simulink model "SimulacionDataReal"  (R2023b)
settings: Solver=ode1be  StartTime=0.0  StopTime=30  FixedStep=0.001  RelTol=1e-3
undefined symbols (not defined in the file): k1, k2, P, W1_0, W2_0
settings Model: Creator=raul  LastModifiedBy=raul
settings OptimizationCC: ReuseModelBlockBuffer=off

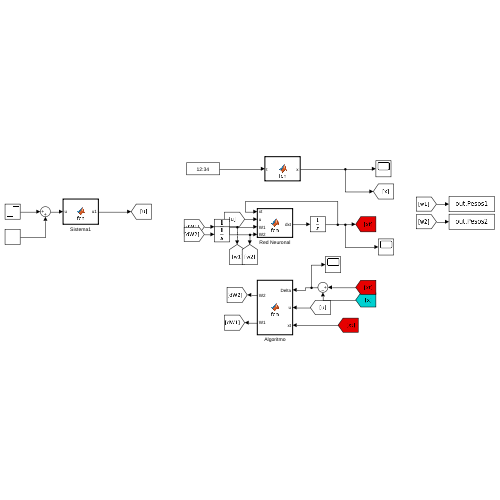
[thumbnail: Simulink's stored preview of the top-level diagram]
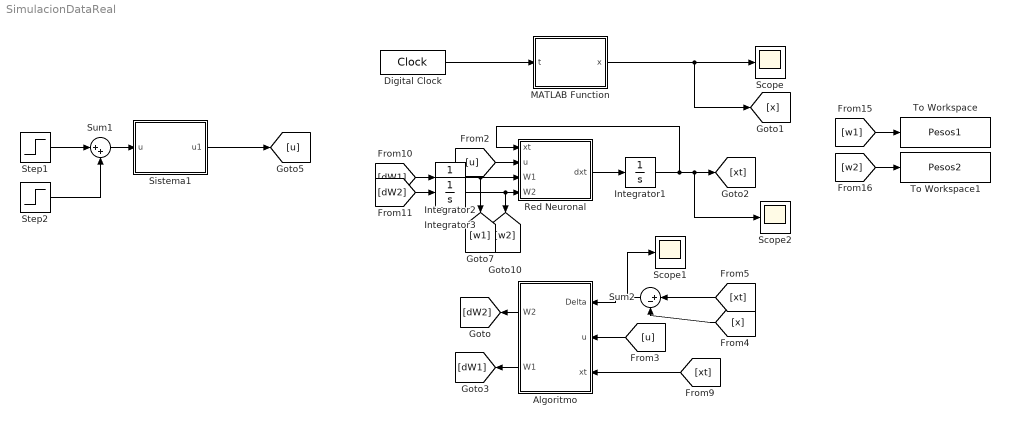
== system SimulacionDataReal ==
  Algoritmo : MATLAB Function  TreatAsAtomicUnit=on
  Digital Clock : DigitalClock  SampleTime=0.01
  Integrator1 : Integrator  InitialCondition=zeros(40,1)
  Integrator2 : Integrator  InitialCondition=W1_0
  Integrator3 : Integrator  InitialCondition=W2_0
  MATLAB Function : MATLAB Function  TreatAsAtomicUnit=on
  Red Neuronal : MATLAB Function  TreatAsAtomicUnit=on
  Scope : Scope
  Scope1 : Scope
  Scope2 : Scope
  Sistema1 : MATLAB Function  TreatAsAtomicUnit=on
  Step1 : Step  Time=13.50  After=10  SampleTime=0
  Step2 : Step  Time=14  After=-10  SampleTime=0
  Sum1 : Sum  Inputs=|++
  Sum2 : Sum  Inputs=|+-
  To Workspace : ToWorkspace  VariableName=Pesos1  SampleTime=-1
  To Workspace1 : ToWorkspace  VariableName=Pesos2  SampleTime=-1
  wires:
  MATLAB Function/1(x) -> [x], Scope/1
  Digital Clock/1 -> MATLAB Function/1(t)
  [x] -> Sum2/2
  Integrator2/1 -> [w1], Red Neuronal/3(W1)
  [dW2] -> Integrator3/1
  [u] -> Algoritmo/2(u)
  Red Neuronal/1(dxt) -> Integrator1/1
  Integrator3/1 -> [w2], Red Neuronal/4(W2)
  Algoritmo/2(W1) -> [dW1]
  Algoritmo/1(W2) -> [dW2]
  [xt] -> Sum2/1
  [u] -> Red Neuronal/2(u)
  Sum2/1 -> Scope1/1, Algoritmo/1(Delta)
  Integrator1/1 -> Scope2/1, [xt], Red Neuronal/1(xt)
  [dW1] -> Integrator2/1
  [xt] -> Algoritmo/3(xt)
  Step2/1 -> Sum1/2
  Step1/1 -> Sum1/1
  Sum1/1 -> Sistema1/1(u)
  Sistema1/1(u1) -> [u]
  [w1] -> To Workspace/1
  [w2] -> To Workspace1/1

== matlab function SimulacionDataReal/Algoritmo ==
  data: W2 output; Delta input; P parameter; u input; W1 output; k1 parameter; k2 parameter; xt input
function [W2,W1] = fcn(Delta,P,u, k1, k2,xt)


W1=-k1*P*Delta*sigmoid(1,xt)';
W2=-k2*P*Delta*u'*phi_function(ones(40,40),xt);



function s = sigmoid(b,x)
   s = 1./(1+exp(-b*x)); 
end

function phi = phi_function(b, x)
    phi=zeros(40,40);
    for i=1:length(x)
        for j=1:length(x)
            sumbx=0;
            for p=1:length(x)
                sumbx=sumbx+(b(i,j)^p)*x(p);
            end
            phi(i,j)=1./(1+exp(-sumbx));
        end
    end
end

end

== matlab function SimulacionDataReal/MATLAB Function ==
  data: x output; t input; Data parameter
function x = fcn(t, Data)

x = Data(:,floor(t*100+1));

== matlab function SimulacionDataReal/Red Neuronal ==
  data: xt input; u input; dxt output; W1 input; A parameter; W2 input
function dxt = fcn(xt, u, W1, A, W2)

dxt = A*xt+W1*sigmoid(1,xt)+W2*ones(40,40)*u;


function s = sigmoid(b,x)
   s = 1./(1+exp(-b*x)); 
end

% function phi = phi_function(b, x)
%     for i=1:length(x)
%         for j=1:length(x)
%             sumbx=0;
%             for p=1:length(x)
%                 sumbx=sumbx+(b(i,j)^p)*x(p);
%             end
%             phi(i,j)=1./(1+exp(-sumbx));
%         end
%     end
% end

end

== matlab function SimulacionDataReal/Sistema1 ==
  data: u1 output; u input
function u1 = fcn(u)%add Bw,w

u1=[0;
    0;
    0;
    0;
    0;
    0;
    0;
    0;
    0;
    0;
    0;
    u;
    0;
    0;
    0;
    0;
    0;
    0;
    0;
    0;
    0;
    0;
    0;
    0;
    0;
    0;
    0;
    0;
    0;
    0;
    0;
    0;
    0;
    0;
    0;
    0;
    0;
    0;
    0;
    0;];
